simulink model "testrig_TwistBeam"  (R2026a)
settings: Solver=ode23t  EnableMultiTasking=on
PostLoadFcn:
  | sm_car_load_vehicle_data(bdroot,'227');
libraries: fl_lib x7, sm_lib x5, Damper_Element x2, Spring_Element x2, nesl_utility x1, Susp_TwistBeam x1
Description:
  | Testrig for Live Axle Suspension
  | 
  | Copyright 2018-2026 The MathWorks, Inc.
settings Model: Creator=smiller  LastModifiedBy=smiller
settings DataIOCC: SignalLoggingName=logsout_testrig_LiveAxle
settings SimscapeCC: SimscapeNominalValues="[{\"value\":\"10\",\"unit\":\"V\"},{\"value\":\"1\",\"unit\":\"A\"},{\"value\":\"10\",\"unit\":\"N*m\"},{\"value\":\"10\",\"unit\":\"bar\"},{\"value\":\"100\",\"unit\":\"kJ/kg\"},{\"value\":\"1\",\"unit\":\"kW\"},{\"value\":\"300\",\"unit\":\"K\"},{\"value\":\"100\",\"unit\":\"cm^3/s\"},{\"value\":\"1\",\"unit\":\"kN\"},{\"value\":\"1\",\"unit\":\"g/cm^3\"},{\"value\":\"1\",\"unit\":\"l\"},{\"value\":\"1\",\"unit\":\"cm^2\"},{\"value\":\"60\",\"unit\":\"Hz\"}]"  SimscapeLogName=simlog_testrig_LiveAxle
settings ConfigurationSet: Description=SimMechanics 2G
settings DiagnosticsConfigSet: SimMechanicsUnconnectedFramePorts=none  SimMechanicsConflictingReferenceFrames=none
settings ExplorerConfigSet: InternalSimMechanicsExplorerSettings="<ExplorerConfiguration><canonicalview>default</canonicalview><AnimationSetting><BasePlaybackSpeed>1.0</BasePlaybackSpeed><PlaybackSpeedFactor>1.0</PlaybackSpeedFactor></AnimationSetting><TilePanel><TileInfo><Tiles Columns=\"2\" Count=\"2\" Rows=\"1\"><Column Weight=\"0.3776\"/><Column Weight=\"0.6224\"/><Row Weight=\"1\"/><Tile Height=\"1\" Width=\"1\" X=\"0\" Y=\"0\"/><Tile Height=\"1\" Width=\"1\" X=\"1\" Y=\"0\"/></Tiles></TileInfo><SceneInfo><SceneViewer><BGColor><R>1</R><G>1</G><B>1</B></BGColor><Camera><DoPerspective>off</DoPerspective><Position><X>0.0871392930886595585</X><Y>-1.26133706249147304</Y><Z>0.386279098991324066</Z></Position><Center><X>0.0871392930886595585</X><Y>-4.702163486358657e-08</Y><Z>0.386279098991324066</Z></Center><Up><X>0</X><Y>-0</Y><Z>1</Z></Up><ViewLimDist>1</ViewLimDist><YLim>0.530243420034647084</YLim><XLim>0.488274346248120994</XLim></Camera></SceneViewer><SceneViewer><BGColor><R>1</R><G>1</G><B>1</B></BGColor><Camera><DoPerspective>off</DoPerspective><Position><X>-0.91676253493676485</X><Y>-0.260210636623209979</Y><Z>0.676523912309515474</Z></Position><Center><X>0.0930148277281637875</X><Y>0.0387248114422125145</Y><Z>0.46547499702495726</Z></Center><Up><X>0.193777372933320258</X><Y>0.0375494918836121183</Y><Z>0.980326662596883613</Z></Up><ViewLimDist>1</ViewLimDist><YLim>0.68444931181206925</YLim><XLim>1.04252993633151081</XLim></Camera></SceneViewer></SceneInfo></TilePanel><MechEditorPanel><Cameras/><GfxPanelCameraMap/><VideoCreator><PlaybackSpeedRatio>1.0</PlaybackSpeedRatio><FrameRate>30</FrameRate><VideoFormat>Motion JPEG AVI</VideoFormat><FrameSize>auto</FrameSize></VideoCreator></MechEditorPanel></ExplorerConfiguration>"

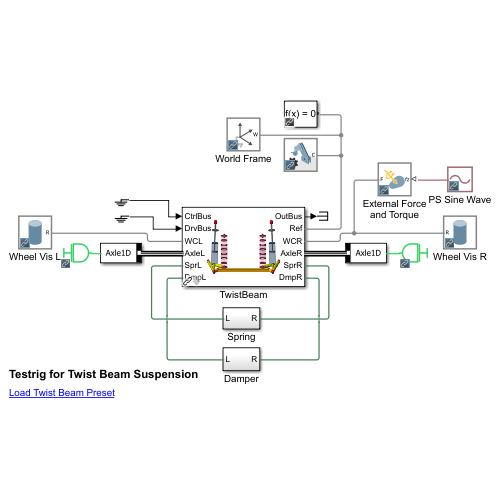
[thumbnail: Simulink's stored preview of the top-level diagram]
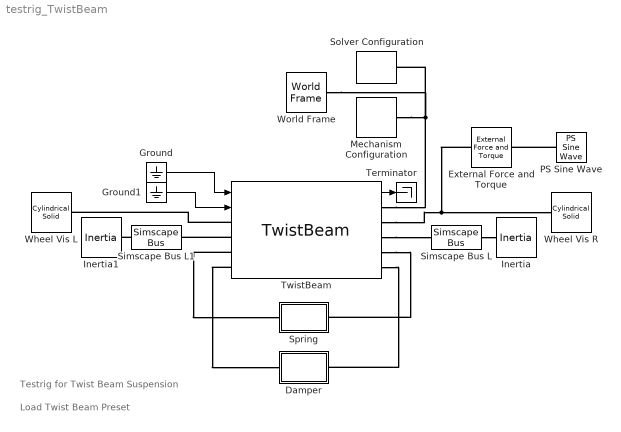
== system testrig_TwistBeam ==
  note: Load Twist Beam Preset
  note: Testrig for Twist Beam Suspension
  Damper : Subsystem
  External Force and Torque : sm_lib/Forces and Torques/External Force and Torque  EnableForceX=off  EnableForceY=off  EnableForceZ=on  EnableForce=off  ForceResolutionFrame=World  EnableTorqueX=off  EnableTorqueY=off  EnableTorqueZ=off  EnableTorque=off  TorqueResolutionFrame=AttachedFrame
  Ground : Ground
  Ground1 : Ground
  Inertia : fl_lib/Mechanical/Rotational Elements/Inertia  inertia=0.01 kg*m^2  num_ports=foundation.enum.numPorts2.one  w_specify=on  w_priority=None  w=0 rad/s  w_nominal_specify=off  w_nominal_value=1  w_nominal_unit=rad/s  t_specify=off  t_priority=None  t=0 N*m  t_nominal_specify=off  t_nominal_value=1  t_nominal_unit=N*m
  Inertia1 : fl_lib/Mechanical/Rotational Elements/Inertia  inertia=0.01 kg*m^2  num_ports=foundation.enum.numPorts2.one  w_specify=on  w_priority=None  w=0 rad/s  w_nominal_specify=off  w_nominal_value=1  w_nominal_unit=rad/s  t_specify=off  t_priority=None  t=0 N*m  t_nominal_specify=off  t_nominal_value=1  t_nominal_unit=N*m
  Mechanism Configuration : sm_lib/Utilities/Mechanism Configuration  UniformGravity=Constant  GravityVector=[0 0 -9.80665]  GravityVectorUnits=m/s^2  LinearizationDelta=0.001  JointModeTransitionNonlinearIterations=2
  PS Sine Wave : fl_lib/Physical Signals/Sources/PS Sine Wave  amplitude=20000  bias=5000  frequency_spec=foundation.enum.frequencySpec.frequencySI  frequency_SI=2 Hz  frequency_angular=1 rad/s  phase=0 rad
  Simscape Bus L : SimscapeBus  HierarchyStrings=Axle1D
  Simscape Bus L1 : SimscapeBus  HierarchyStrings=Axle1D
  Solver Configuration : nesl_utility/Solver Configuration  PhysicalDomain=network_engine_domain  SubClassName=solver  LeftPortType=input  RightPortType=generic  Tones=[]  Harmonics=[]  SimulateNoise=off  Profile=off  UseLocalSampling=off  EnableSwitchedLinearOptims=on  FrequencyDomain=off  UseCCode=off  RelTol=0.001  AbsTol=1e-06  MinStep=1e-09  ToWorkspace=off  RevertToSquareIcSolve=off  NumHomotopyIterations=100  PhasorMode=off  PhasorModeNumHarmonics=1  ConsistencySolver=NEWTON_FTOL  CanonicalOrdering=UNORDERED  OptimizeIntermediates=UNOPTIMIZED  IndexReductionMethod=DerivativeReplacement  DoDC=off  ResidualTolerance=1e-09  ConsistencyTolSource=GLOBAL  ConsistencyAbsTol=0.001  ConsistencyRelTol=0.001  ConsistencyTolFactor=0.001  UseLocalSolver=off  LocalSolverChoice=NE_BACKWARD_EULER_ADVANCER  ResolveIndetEquations=on  FunctionEvalNumThread=1  LocalSolverSampleTime=0.001  DoFixedCost=off  MaxNonlinIter=3  MaxModeIter=2  ComputeImpulses=off  ImpulseIterations=2  LinearAlgebra=Sparse  LinearAlgebraNumThread=0  EquationFormulation=NE_TIME_EF  DelaysMemoryBudget=1024  AutomaticFiltering=on  FilteringTimeConstant=0.001  PartitionStorageMethod=AS_NEEDED  PartitionMemoryBudget=1024  PartitionMethod=FAST  MultibodyUseLocalSolver=off  MultibodyLocalSolverChoice=ODE1  MultibodyLocalSolverSampleTime=0.001
  Spring : Subsystem
  Terminator : Terminator
  TwistBeam : Susp_TwistBeam/TwistBeam  VariantControl=LiveAxle  Init=Init.Axle2  hp_arm=Vehicle.Chassis.SuspA2.TwistBeam.TrailingArm.sBody.Value  hp_dmp_top=Vehicle.Chassis.SuspA2.TwistBeam.Damper.sTop.Value  hp_dmp_bot=Vehicle.Chassis.SuspA2.TwistBeam.Damper.sBottom.Value  hp_spr_top=Vehicle.Chassis.SuspA2.TwistBeam.Spring.sTop.Value  hp_spr_bot=Vehicle.Chassis.SuspA2.TwistBeam.Spring.sBottom.Value  hp_beam=Vehicle.Chassis.SuspA2.TwistBeam.Beam.sOutboard.Value  hp_whl_ctr=Vehicle.Chassis.SuspA2.TwistBeam.TrailingArm.sWheelCentre.Value  Arm_to_Subframe=Vehicle.Chassis.SuspA2.TwistBeam.Arm_to_Subframe  Damper_to_Subframe=Vehicle.Chassis.SuspA2.TwistBeam.Damper_to_Subframe  Damper_to_Arm=Vehicle.Chassis.SuspA2.TwistBeam.Damper_to_Arm  arm_mass=Vehicle.Chassis.SuspA2.TwistBeam.TrailingArm.m.Value  axle_mass=Vehicle.Chassis.SuspA2.TwistBeam.TrailingArm.mAxle.Value  axle_len=Vehicle.Chassis.SuspA2.TwistBeam.TrailingArm.xAxle.Value  axle_whlc_to_bearing=Vehicle.Chassis.SuspA2.TwistBeam.TrailingArm.xWCtoBearing.Value  beam_rho=Vehicle.Chassis.SuspA2.TwistBeam.Beam.density.Value  beam_E=Vehicle.Chassis.SuspA2.TwistBeam.Beam.E.Value  beam_nu=Vehicle.Chassis.SuspA2.TwistBeam.Beam.nu.Value  beam_zeta=Vehicle.Chassis.SuspA2.TwistBeam.Beam.zDamping.Value  xc_x=Vehicle.Chassis.SuspA2.TwistBeam.Beam.xcX.Value  xc_z=Vehicle.Chassis.SuspA2.TwistBeam.Beam.xcZ.Value  beam_numElements=Vehicle.Chassis.SuspA2.TwistBeam.Beam.numElements.Value  opc_beam=Visual.part.opc  clr_beam=Visual.clr.orangedark  radius_axle=Visual.Axle.rad  clr_axle=Visual.Axle.clr  opc_axle=Visual.part.opc  clr_upr=Visual.UpperArm.clr  opc_upr=Visual.part.opc  piston_mass=Vehicle.Chassis.SuspA2.TwistBeam.Damper.mPiston.Value  cyl_mass=Vehicle.Chassis.SuspA2.TwistBeam.Damper.mCylinder.Value  damper_xmax=Vehicle.Chassis.SuspA2.TwistBeam.Endstop.xMax.Value  damper_xmin=Vehicle.Chassis.SuspA2.TwistBeam.Endstop.xMin.Value  spring_mass=Vehicle.Chassis.SuspA2.TwistBeam.Spring.m.Value
  Wheel Vis L : sm_lib/Body Elements/Cylindrical Solid  CylinderRadius=0.3  CylinderRadiusUnits=m  CylinderLength=0.1  CylinderLengthUnits=m  ExportEntireGeometry=off  InertiaType=CalculateFromGeometry  BasedOnType=Density  Density=1000  DensityUnits=kg/m^3  Mass=1  MassUnits=kg  CenterOfMass=[0 0 0]  CenterOfMassUnits=m  MomentsOfInertia=[1 1 1]  MomentsOfInertiaUnits=kg*m^2  ProductsOfInertia=[0 0 0]  ProductsOfInertiaUnits=kg*m^2  GraphicType=FromGeometry  MarkerShape=Sphere  MarkerSize=10  GraphicVisPropType=SimpleVisualProperties  GraphicDiffuseColor=[0.5 0.5 0.5]  GraphicOpacity=0.3  GraphicSpecularColor=[0.5 0.5 0.5 1.0]  GraphicAmbientColor=[0.15 0.15 0.15 1.0]  GraphicEmissiveColor=[0.0 0.0 0.0 1.0]  GraphicShininess=75  DoExposeReferenceFrame=on  SerializedFrames=<Frames/>
  Wheel Vis R : sm_lib/Body Elements/Cylindrical Solid  CylinderRadius=0.3  CylinderRadiusUnits=m  CylinderLength=0.1  CylinderLengthUnits=m  ExportEntireGeometry=off  InertiaType=CalculateFromGeometry  BasedOnType=Density  Density=1000  DensityUnits=kg/m^3  Mass=1  MassUnits=kg  CenterOfMass=[0 0 0]  CenterOfMassUnits=m  MomentsOfInertia=[1 1 1]  MomentsOfInertiaUnits=kg*m^2  ProductsOfInertia=[0 0 0]  ProductsOfInertiaUnits=kg*m^2  GraphicType=FromGeometry  MarkerShape=Sphere  MarkerSize=10  GraphicVisPropType=SimpleVisualProperties  GraphicDiffuseColor=[0.5 0.5 0.5]  GraphicOpacity=0.3  GraphicSpecularColor=[0.5 0.5 0.5 1.0]  GraphicAmbientColor=[0.15 0.15 0.15 1.0]  GraphicEmissiveColor=[0.0 0.0 0.0 1.0]  GraphicShininess=75  DoExposeReferenceFrame=on  SerializedFrames=<Frames/>
  World Frame : sm_lib/Frames and Transforms/World Frame
  wires:
  Ground/1 -> TwistBeam/1
  Ground1/1 -> TwistBeam/2
  TwistBeam/1 -> Terminator/1
  connections:
  Mechanism Configuration/RConn1 -- World Frame/RConn1 -- Solver Configuration/RConn1 -- TwistBeam/RConn1
  TwistBeam/LConn1 -- Wheel Vis L/RConn1
  Simscape Bus L/LConn1 -- Inertia/LConn1
  TwistBeam/LConn3 -- Spring/LConn1
  TwistBeam/RConn4 -- Spring/RConn1
  TwistBeam/RConn3 -- Simscape Bus L/RConn1
  Simscape Bus L1/LConn1 -- Inertia1/LConn1
  TwistBeam/LConn2 -- Simscape Bus L1/RConn1
  TwistBeam/LConn4 -- Damper/LConn1
  External Force and Torque/RConn1 -- Wheel Vis R/RConn1 -- TwistBeam/RConn2
  TwistBeam/RConn5 -- Damper/RConn1
  PS Sine Wave/RConn1 -- External Force and Torque/LConn1

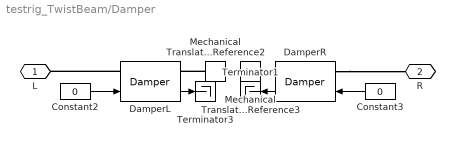
== system testrig_TwistBeam/Damper ==
  Constant2 : Constant  Value=0
  Constant3 : Constant  Value=0
  DamperL : Damper_Element/Damper  VariantControl=Variant1  LabelModeActiveChoice=Linear  Damper=Vehicle.Chassis.Damper.Axle2  VariantLabel=Vehicle.Chassis.Damper.Axle2.class.Value
      settings: AttributesFormatString=%<ActiveVariant>
  DamperR : Damper_Element/Damper  VariantControl=Variant1  LabelModeActiveChoice=Linear  Damper=Vehicle.Chassis.Damper.Axle2  VariantLabel=Vehicle.Chassis.Damper.Axle2.class.Value
      settings: AttributesFormatString=%<ActiveVariant>
  Mechanical Translational Reference2 : fl_lib/Mechanical/Translational Elements/Mechanical Translational Reference
  Mechanical Translational Reference3 : fl_lib/Mechanical/Translational Elements/Mechanical Translational Reference
  Terminator1 : Terminator
  Terminator3 : Terminator
  L : PMIOPort  Side=Left
  R : PMIOPort  Port=2  Side=Right
  wires:
  DamperR/1 -> Terminator1/1
  Constant3/1 -> DamperR/1
  Constant2/1 -> DamperL/1
  DamperL/1 -> Terminator3/1
  connections:
  DamperL/LConn1 -- L/RConn1
  Mechanical Translational Reference2/LConn1 -- DamperL/RConn1
  Mechanical Translational Reference3/LConn1 -- DamperR/RConn1
  DamperR/LConn1 -- R/RConn1

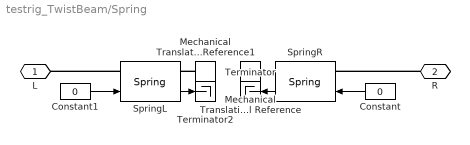
== system testrig_TwistBeam/Spring ==
  Constant : Constant  Value=0
  Constant1 : Constant  Value=0
  Mechanical Translational Reference : fl_lib/Mechanical/Translational Elements/Mechanical Translational Reference
  Mechanical Translational Reference1 : fl_lib/Mechanical/Translational Elements/Mechanical Translational Reference
  SpringL : Spring_Element/Spring  VariantControl=Variant1  LabelModeActiveChoice=Linear  Spring=Vehicle.Chassis.Spring.Axle2  VariantLabel=Vehicle.Chassis.Spring.Axle2.class.Value
      settings: AttributesFormatString=%<ActiveVariant>
  SpringR : Spring_Element/Spring  VariantControl=Variant1  LabelModeActiveChoice=Linear  Spring=Vehicle.Chassis.Spring.Axle1  VariantLabel=Vehicle.Chassis.Spring.Axle1.class.Value
      settings: AttributesFormatString=%<ActiveVariant>
  Terminator : Terminator
  Terminator2 : Terminator
  L : PMIOPort  Side=Left
  R : PMIOPort  Port=2  Side=Right
  wires:
  SpringL/1 -> Terminator2/1
  Constant1/1 -> SpringL/1
  SpringR/1 -> Terminator/1
  Constant/1 -> SpringR/1
  connections:
  Mechanical Translational Reference1/LConn1 -- SpringL/RConn1
  Mechanical Translational Reference/LConn1 -- SpringR/RConn1
  R/RConn1 -- SpringR/LConn1
  SpringL/LConn1 -- L/RConn1
